simulink model "miniLab_AD_test"  (Simulink 4.00)
settings: Solver=FixedStepDiscrete  SolverMode=SingleTasking  StartTime=0.0  StopTime=3  FixedStep=0.05  RelTol=1e-3
libraries: rt_sync_lib x1
settings Model: LastModifiedBy=bsaunder

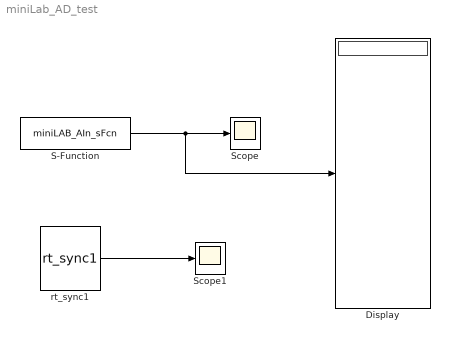
== system miniLab_AD_test ==
  Display : Display
      settings: Format=short
  S-Function : S-Function  FunctionName=miniLAB_AIn_sFcn  Parameters=0.05, [0 1 2 3]  PortCounts=[]  SFunctionModules=''
  Scope : Scope
      settings: TimeRange=3  YMin=-1  YMax=6  SaveToWorkspace=off  SaveName=ScopeData  LimitDataPoints=on  MaxDataPoints=5000
  Scope1 : Scope
      settings: TimeRange=3  YMin=-1  YMax=6  SaveToWorkspace=off  LimitDataPoints=on  MaxDataPoints=5000
  rt_sync1 : rt_sync_lib/rt_sync1  Ts=0.05
  wires:
  S-Function/1 -> Scope/1, Display/1
  rt_sync1/1 -> Scope1/1
